simulink model "pendulum_ctrl_sim_1"  (R2023a)
settings: Solver=VariableStepAuto  StartTime=0.0  StopTime=Tf_1  MaxStep=MaxStep  RelTol=RelTol
values from neighbouring files (symbols this model uses):
  b = 0.05    [p60_pendulum_control.m]
  g = 9.81    [p60_pendulum_control.m]
  l = 0.3    [p60_pendulum_control.m]
  M = 0.5    [p60_pendulum_control.m]
  R_u = 0.75    [p60_pendulum_control.m]
  theta_star_u = 2*pi/3    (= 2.09439510239)    [p60_pendulum_control.m]
  x0_1 = [i; j]    [p60_pendulum_control.m]
settings Model: Creator=alessandro  LastModifiedBy=admin
settings OptimizationCC: ReuseModelBlockBuffer=off

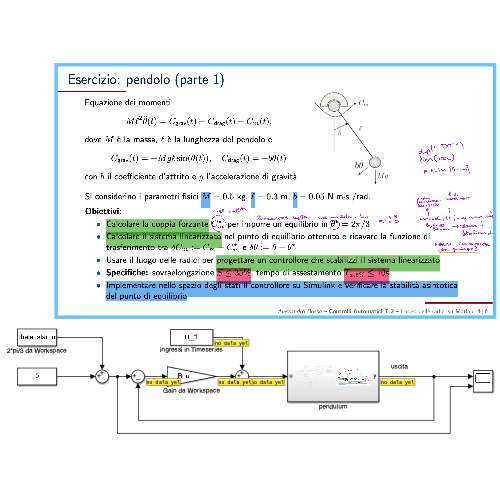
[thumbnail: Simulink's stored preview of the top-level diagram]
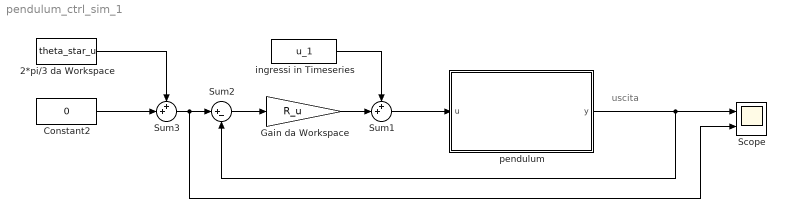
== system pendulum_ctrl_sim_1 ==
  note: uscita
  2*pi/3 da Workspace : Constant  Value=theta_star_u
  Constant2 : Constant  Value=0
  Gain da Workspace : Gain  Gain=R_u
  Scope : Scope  NumInputPorts=2
  Sum1 : Sum  Inputs=++|
  Sum2 : Sum  Inputs=|+-
  Sum3 : Sum  Inputs=++|
  ingressi in Timeseries : FromWorkspace  VariableName=u_1
  pendulum : Subsystem
  wires:
  pendulum/1(y) -> Scope/1, Sum2/2
  2*pi/3 da Workspace/1 -> Sum3/1
  Sum2/1 -> Gain da Workspace/1
  ingressi in Timeseries/1 -> Sum1/1
  Gain da Workspace/1 -> Sum1/2
  Sum1/1 -> pendulum/1(u)
  Sum3/1 -> Scope/2, Sum2/1
  Constant2/1 -> Sum3/2

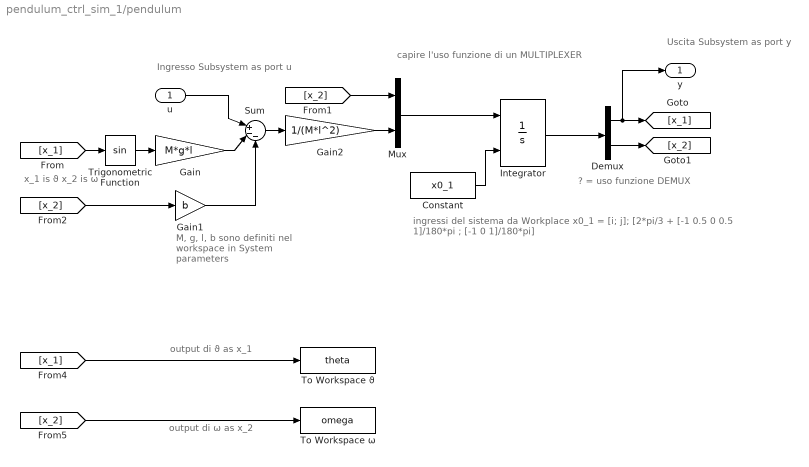
== system pendulum_ctrl_sim_1/pendulum ==
  note: Uscita Subsystem
      | as port y
  note: Ingresso Subsystem
      | as port u
  note: ? = uso funzione DEMUX
  note: capire l'uso funzione di un MULTIPLEXER
  note: x_1 is ϑ
      |
      | x_2 is ω
  note: output di ϑ as x_1
  note: output di ω as x_2
  note: ingressi del sistema
      | da Workplace
      | x0_1 = [i; j];
      | [2*pi/3 + [-1 0.5 0 0.5 1]/180*pi ; [-1 0 1]/180*pi]
  note: M, g, l, b
      | sono definiti
      | nel workspace in
      | System parameters
  u : Inport
  Constant : Constant  Value=x0_1
  Demux : Demux  Outputs=2
  Gain : Gain  Gain=M*g*l
  Gain1 : Gain  Gain=b
  Gain2 : Gain  Gain=1/(M*l^2)
  Integrator : Integrator  InitialConditionSource=external
  Mux : Mux  Inputs=2
  Sum : Sum  Inputs=|+--
  To Workspace ω : ToWorkspace  VariableName=omega  SaveFormat=Timeseries  SampleTime=-1
  To Workspace ϑ : ToWorkspace  VariableName=theta  SaveFormat=Timeseries  SampleTime=-1
  Trigonometric Function : Trigonometry
  y : Outport
  wires:
  [x_2] -> Gain1/1
  [x_1] -> To Workspace ϑ/1
  Mux/1 -> Integrator/1
  Sum/1 -> Gain2/1
  Demux/2 -> [x_2]
  Integrator/1 -> Demux/1
  [x_2] -> To Workspace ω/1
  Demux/1 -> y/1, [x_1]
  Gain1/1 -> Sum/3
  Gain2/1 -> Mux/2
  [x_1] -> Trigonometric Function/1
  Constant/1 -> Integrator/2
  Gain/1 -> Sum/2
  Trigonometric Function/1 -> Gain/1
  [x_2] -> Mux/1
  u/1 -> Sum/1
